simulink model "fullSystemModel"  (R2018a)
settings: Solver=ode3  StartTime=0.0  StopTime=1000  FixedStep=1  MinStep=1e-8  RelTol=1e-8
undefined symbols (not defined in the file or in its folder): DiscIntNeverNeededParam
libraries: BupSimulinkLibraries x32, simulink_extras x22, simulink x2, SignalEditorBlockLib x2
(part 2 of 3)

== system fullSystemModel/Easy_reg1/DataAnalyzer/InternalTrackingCourse ==
  Position : Inport  OutDataTypeStr=double  PortDimensions=3
  Azimuth : BupSimulinkLibraries/Azimuth
  Bearing : BupSimulinkLibraries/Bearing
  Display : Display
  Display1 : Display
  LastPos : Delay  DelayLength=1
  Manual Switch2 : ManualSwitch
  Radians to Degrees1 : simulink_extras/Transformations/Radians to Degrees
  Radians to Degrees2 : simulink_extras/Transformations/Radians to Degrees
  Scope1 : Scope  NumInputPorts=2
  Scope8 : Scope
  Scope9 : Scope
  Course : Outport  OutDataTypeStr=double  PortDimensions=1
  wires:
  Bearing/1 -> Manual Switch2/1, Display/1, Radians to Degrees1/1, Scope8/1
  Azimuth/1 -> Manual Switch2/2, Scope9/1, Radians to Degrees2/1, Display1/1
  Manual Switch2/1 -> Course/1
  LastPos/1 -> Azimuth/2, Bearing/2
  Position/1 -> LastPos/1, Bearing/1, Azimuth/1
  Radians to Degrees1/1 -> Scope1/1
  Radians to Degrees2/1 -> Scope1/2

== system fullSystemModel/Easy_reg1/DataAnalyzer/InternalTrackingSpeed ==
  Position : Inport
  Constant : Constant
  GPSVelocity : BupSimulinkLibraries/GPSVelocity
  LastPos1 : Delay  DelayLength=1
  ProjectionSpeed : BupSimulinkLibraries/ProjectionSpeed
  Hor_Velocity : Outport
  Ver_Velocity : Outport  Port=2
  wires:
  LastPos1/1 -> GPSVelocity/2
  ProjectionSpeed/2 -> Ver_Velocity/1
  Position/1 -> LastPos1/1, GPSVelocity/1
  ProjectionSpeed/1 -> Hor_Velocity/1
  GPSVelocity/1 -> ProjectionSpeed/1
  GPSVelocity/2 -> ProjectionSpeed/2
  GPSVelocity/3 -> ProjectionSpeed/3
  Constant/1 -> GPSVelocity/3

== system fullSystemModel/Easy_reg1/Targeting/Roughening ==
  Input : Inport
  DeadZone : BupSimulinkLibraries/DeadZone
  Gain : Gain  Gain=0.1
  Gain1 : Gain  Gain=10
  Manual Switch : ManualSwitch  CurrentSetting=0
  Rounding Function : Rounding
  Scope : Scope  NumInputPorts=3
  Output : Outport
  wires:
  Input/1 -> Scope/1, Gain/1
  Gain/1 -> Rounding Function/1
  Rounding Function/1 -> Gain1/1
  Gain1/1 -> Manual Switch/2, DeadZone/1, Scope/2
  DeadZone/1 -> Manual Switch/1, Scope/3
  Manual Switch/1 -> Output/1

== system fullSystemModel/Plant/GNSS/InternalTrackingCourse ==
  Position : Inport  OutDataTypeStr=double  PortDimensions=3
  Azimuth : BupSimulinkLibraries/Azimuth
  Bearing : BupSimulinkLibraries/Bearing
  Display : Display
  Display1 : Display
  LastPos : Memory  InheritSampleTime=on
  Manual Switch2 : ManualSwitch  CurrentSetting=0
  Scope1 : Scope  NumInputPorts=2
  Scope8 : Scope
  Scope9 : Scope
  Course : Outport  OutDataTypeStr=double  PortDimensions=1
  wires:
  Bearing/1 -> Scope1/1, Display/1, Manual Switch2/1, Scope8/1
  Azimuth/1 -> Display1/1, Scope1/2, Manual Switch2/2, Scope9/1
  Manual Switch2/1 -> Course/1
  LastPos/1 -> Azimuth/2, Bearing/2
  Position/1 -> LastPos/1, Bearing/1, Azimuth/1

== system fullSystemModel/Plant/GNSS/InternalTrackingCourse1 ==
  Position : Inport  OutDataTypeStr=double  PortDimensions=3
  Azimuth : BupSimulinkLibraries/Azimuth
  Bearing : BupSimulinkLibraries/Bearing
  Display : Display
  Display1 : Display
  LastPos : Memory  InheritSampleTime=on
  Manual Switch2 : ManualSwitch  CurrentSetting=0
  Scope1 : Scope  NumInputPorts=2
  Scope8 : Scope
  Scope9 : Scope
  Course : Outport  OutDataTypeStr=double  PortDimensions=1
  wires:
  Bearing/1 -> Scope1/1, Display/1, Manual Switch2/1, Scope8/1
  Azimuth/1 -> Display1/1, Scope1/2, Manual Switch2/2, Scope9/1
  Manual Switch2/1 -> Course/1
  LastPos/1 -> Azimuth/2, Bearing/2
  Position/1 -> LastPos/1, Bearing/1, Azimuth/1

== system fullSystemModel/Plant/GNSS/TrackingSpeed ==
  Position : Inport
  Constant : Constant
  GPSVelocity : BupSimulinkLibraries/GPSVelocity
  LastPos : Memory  InheritSampleTime=on  LinearizeAsDelay=on
  Vel_Latitude : Outport
  Vel_Longitude : Outport  Port=2
  Vel_Altitude : Outport  Port=3
  wires:
  LastPos/1 -> GPSVelocity/2
  Position/1 -> GPSVelocity/1, LastPos/1
  Constant/1 -> GPSVelocity/3
  GPSVelocity/3 -> Vel_Altitude/1
  GPSVelocity/2 -> Vel_Longitude/1
  GPSVelocity/1 -> Vel_Latitude/1

== system fullSystemModel/Plant/GNSS/Transformation ==
  InitialPos : Inport
  x : Inport  Port=2
  y : Inport  Port=3
  Bus Selector : BusSelector  OutputSignals=Initial_lat,Initial_lon
  Degrees to Radians : simulink_extras/Transformations/Degrees to Radians
  Divide : Product  Inputs=*/
  Gain : Gain  Gain=1/1000
  Gain1 : Gain  Gain=1/1000
  Gain5 : Gain  Gain=360/40000
  Gain6 : Gain  Gain=360/40000
  Sum : Sum  Inputs=++|
  Sum1 : Sum  Inputs=|++
  Trigonometric Function2 : Trigonometry  Operator=cos
  Latitude : Outport
  Longitude : Outport  Port=2
  wires:
  Divide/1 -> Sum1/1
  Gain5/1 -> Divide/1
  y/1 -> Gain1/1
  Gain6/1 -> Sum/1
  x/1 -> Gain/1
  Trigonometric Function2/1 -> Divide/2
  Degrees to Radians/1 -> Trigonometric Function2/1
  Gain/1 -> Gain5/1
  Gain1/1 -> Gain6/1
  InitialPos/1 -> Bus Selector/1
  Bus Selector/1 -> Sum/2  "<Initial_lat>"
  Bus Selector/2 -> Sum1/2  "<Initial_lon>"
  Sum/1 -> Degrees to Radians/1, Latitude/1
  Sum1/1 -> Longitude/1

== system fullSystemModel/Plant/GNSS/Transformation1 ==
  InitialPos : Inport
  x : Inport  Port=2
  y : Inport  Port=3
  Bus Selector : BusSelector  OutputSignals=Initial_lat,Initial_lon
  Degrees to Radians : simulink_extras/Transformations/Degrees to Radians
  Divide : Product  Inputs=*/
  Gain : Gain  Gain=1/1000
  Gain1 : Gain  Gain=1/1000
  Gain5 : Gain  Gain=360/40000
  Gain6 : Gain  Gain=360/40000
  Sum : Sum  Inputs=++|
  Sum1 : Sum  Inputs=|++
  Trigonometric Function2 : Trigonometry  Operator=cos
  Latitude : Outport
  Longitude : Outport  Port=2
  wires:
  Sum1/1 -> Longitude/1
  Sum/1 -> Latitude/1, Degrees to Radians/1
  Bus Selector/2 -> Sum1/2  "<Initial_lon>"
  Bus Selector/1 -> Sum/2  "<Initial_lat>"
  InitialPos/1 -> Bus Selector/1
  Gain1/1 -> Gain6/1
  Gain/1 -> Gain5/1
  Degrees to Radians/1 -> Trigonometric Function2/1
  Trigonometric Function2/1 -> Divide/2
  x/1 -> Gain/1
  Gain6/1 -> Sum/1
  y/1 -> Gain1/1
  Gain5/1 -> Divide/1
  Divide/1 -> Sum1/1

== system fullSystemModel/Plant/WindCreator/RotateOnNorth ==
  AbsoluteAngle : Inport
  Constant : Constant  Value=90
  Gain : Gain  Gain=-1
  Sum3 : Sum  Inputs=|+-
  OrientedOnNorth : Outport
  wires:
  AbsoluteAngle/1 -> Sum3/1
  Constant/1 -> Sum3/2
  Sum3/1 -> Gain/1
  Gain/1 -> OrientedOnNorth/1

== system fullSystemModel/flightController/DataAnalyzer/InternalTrackingCourse ==
  Position : Inport  OutDataTypeStr=double  PortDimensions=3
  Azimuth : BupSimulinkLibraries/Azimuth
  Bearing : BupSimulinkLibraries/Bearing
  Display : Display
  Display1 : Display
  LastPos : Delay  DelayLength=1
  Manual Switch2 : ManualSwitch
  Radians to Degrees1 : simulink_extras/Transformations/Radians to Degrees
  Radians to Degrees2 : simulink_extras/Transformations/Radians to Degrees
  Scope1 : Scope  NumInputPorts=2
  Scope8 : Scope
  Scope9 : Scope
  Course : Outport  OutDataTypeStr=double  PortDimensions=1
  wires:
  Bearing/1 -> Manual Switch2/1, Display/1, Radians to Degrees1/1, Scope8/1
  Azimuth/1 -> Manual Switch2/2, Scope9/1, Radians to Degrees2/1, Display1/1
  Manual Switch2/1 -> Course/1
  LastPos/1 -> Azimuth/2, Bearing/2
  Position/1 -> LastPos/1, Bearing/1, Azimuth/1
  Radians to Degrees1/1 -> Scope1/1
  Radians to Degrees2/1 -> Scope1/2

== system fullSystemModel/flightController/DataAnalyzer/InternalTrackingSpeed ==
  Position : Inport
  ExternalVelocity : Inport  Port=2
  Bus Selector1 : BusSelector  OutputSignals=gpsVelocity:latitude,gpsVelocity:longitude,gpsVelocity:altitude
  Constant : Constant
  GPSVelocity : BupSimulinkLibraries/GPSVelocity
  LastPos1 : Delay  DelayLength=1
  ProjectionSpeed : BupSimulinkLibraries/ProjectionSpeed
  Terminator : Terminator
  Terminator1 : Terminator
  Terminator2 : Terminator
  Hor_Velocity : Outport
  Ver_Velocity : Outport  Port=2
  wires:
  LastPos1/1 -> GPSVelocity/2
  ProjectionSpeed/2 -> Ver_Velocity/1
  Position/1 -> LastPos1/1, GPSVelocity/1
  ProjectionSpeed/1 -> Hor_Velocity/1
  Constant/1 -> GPSVelocity/3
  ExternalVelocity/1 -> Bus Selector1/1
  Bus Selector1/1 -> ProjectionSpeed/1  "<gpsVelocity:latitude>"
  Bus Selector1/2 -> ProjectionSpeed/2  "<gpsVelocity:longitude>"
  Bus Selector1/3 -> ProjectionSpeed/3  "<gpsVelocity:altitude>"
  GPSVelocity/1 -> Terminator/1
  GPSVelocity/2 -> Terminator1/1
  GPSVelocity/3 -> Terminator2/1

== system fullSystemModel/flightController/Targeting/Roughening ==
  Input : Inport
  DeadZone : BupSimulinkLibraries/DeadZone
  Gain : Gain  Gain=0.1
  Gain1 : Gain  Gain=10
  Manual Switch : ManualSwitch
  Rounding Function : Rounding
  Scope : Scope  NumInputPorts=3
  Output : Outport
  wires:
  Gain/1 -> Rounding Function/1
  Rounding Function/1 -> Gain1/1
  Gain1/1 -> Manual Switch/2, DeadZone/1, Scope/2
  DeadZone/1 -> Manual Switch/1, Scope/3
  Manual Switch/1 -> Output/1
  Input/1 -> Scope/1, Gain/1

== stateflow chart fullSystemModel/flightController/LogicController ==
  state Timer [parallel]
    entry:
    time = 0;
    BimSupply.timeout = 0;
    Control.Flight.StepAngle.timeout = 0;
    during:
    time = time + 1;
    BimSupply.timeout = TimeoutDecrement(BimSupply.timeout);
    Control.Flight.StepAngle.timeout = TimeoutDecrement(Control.Flight.StepAngle.timeout);
    settings: executionOrder=1
  state Control [parallel]
    % Основной цикл задач
    settings: executionOrder=2
    state Init % Производим планирование путевых точек для сброса высоты
      entry:
      targetPoint = touchdownPoint;
      %[Flight.Angle.Point1, Flight.Angle.Point2] = AngleManCreator(currentPoint, touchdownPoint, AngleManevr);
      %[Flight.Box.LUPoint, Flight.Box.LDPoint, Flight.Box.RUPoint, Flight.Box.RDPoint] = BOXCreator(touchdownPoint, BoxSize);
      Control.Flight.StepAngle.justReturnedHere = false;
      Control.Flight.StepAngle.waiting = true;
      initialPoint = currentPoint;
      touchdownPoint_Offset = [0;0;0];
    state TDP_Only % Режим прицеливания на TDP
      targetPoint = touchdownPoint;
      courseToTargetPoint = Azimut(targetPoint, currentPoint);
      %courseToTargetPoint = Heading(targetPoint, currentPoint, 0);
      desiredCourse = courseToTargetPoint;
    state Flight % Режим полета по точкам
      courseToTargetPoint = Azimut(targetPoint + touchdownPoint_Offset, currentPoint);
      %courseToTargetPoint = Heading(targetPoint + touchdownPoint_Offset, currentPoint, 0);
      desiredCourse = courseToTargetPoint;
      (history)
      state StepAngle
        coeff = nonlinearCoefficientFunction;
        timeDifference = timeVertical - timeHorizontal;
        state Right
          entry:
          timeout = uint32((timeDifference)*coeff)
          waiting = false;
          justReturnedHere = false;
          BimSupply.wantEnable;
          during:
          desiredCourse = Angle2Course(desiredCourse+AngleManevr);
          exit:
          if wherePoint(initialPoint, touchdownPoint, currentPoint) == -1
          side = false;
          else
          side = true;
          end
        state Wait
          entry:
          BimSupply.wantEnable
          waiting = true;
          justReturnedHere = true;
          exit:
          centralCourse = course;
        state Left
          entry:
          timeout = uint32((timeDifference)*coeff)
          waiting = false;
          justReturnedHere = false;
          BimSupply.wantEnable;
          during:
          desiredCourse = Angle2Course(desiredCourse-AngleManevr);
          exit:
          side = true;
          if wherePoint(initialPoint, touchdownPoint, currentPoint) == 1
          side = true;
          else
          side = false;
          end
        state Exit
        Right -> (junction 627) [order 2] : [errorCourseLimit]
            | {timeout = AngleTimeout/2;}
        Right -> (junction 627) [order 1] : [timeout == 0]
            | {timeout = AngleTimeout;}
        (default) -> Wait : {timeout = 15;}
        (junction 627) -> Wait
        Right -> (junction 627) [commented out] : Final
            | {timeout = AngleTimeout/2;}
        (junction 583) -> Right [order 1] : [side]
        Wait -> (junction 583) [order 1] : [(timeDifference) > 1  && timeout == 0]
        (junction 583) -> Left [order 2] : [~side]
        (default) -> Wait [commented out]
        Wait -> Exit [order 2] : [distanceToTarget < 500]
        Left -> (junction 624) [order 1] : [timeout == 0]
            | {timeout = AngleTimeout;}
        (junction 624) -> Wait
        Left -> (junction 624) [commented out] : Final
            | {timeout = AngleTimeout/2;}
        Left -> (junction 624) [order 2] : [errorCourseLimit]
            | {timeout = AngleTimeout/2;}
      state Angle % Режим углового манёвра [commented out]
        entry:
        targetPoint = EntryAngleMan (Point1, Point2, currentPoint, course);
      state Box [commented out]
        % LU - Нацеливание на верхний левый угол "коробки"
        % LD - Нацеливание на нижний левый угол "коробки"
        % RD - Нацеливание на нижний правый угол "коробки"
        % RU - Нацеливание на верхний правый угол "коробки"
        (history)
        state Init [commented out]
          BoxEntry = VerticeSelect(currentPoint, LUPoint, LDPoint, RUPoint, RDPoint);
        state RU [commented out]
          entry:
          targetPoint = RUPoint;
        state LU [commented out]
          entry:
          targetPoint = LUPoint;
        state LD [commented out]
          entry:
          targetPoint = LDPoint;
        state RD [commented out]
          entry:
          targetPoint = RDPoint;
        (default) -> Control.Flight.Box.Init [commented out]
        Control.Flight.Box.Init -> (junction 247) [commented out]
        (junction 247) -> RU [commented out] : [BoxEntry == 3]
        RU -> LU [commented out] : NextStage
        (junction 247) -> LU [commented out] : [BoxEntry == 1]
        LU -> LD [commented out] : NextStage
        RD -> RU [commented out] : NextStage
        (junction 247) -> RD [commented out] : [BoxEntry == 4]
        (junction 247) -> LD [commented out] : [BoxEntry == 2]
        LD -> RD [commented out] : NextStage
      state Final [commented out]
        % Состояние последнего манёвра
        % Цель которого выйти на заданную
        % точку приземления
        BimSupply.wantEnable;
        targetPoint = touchdownPoint
      note: Разрешаем обратные переходы,
          | но с таймаутом, чтобы избежать
          | лишних  переключений
      (default) -> (junction 265)
      (junction 265) -> StepAngle : [Mode == 2]
      (junction 265) -> Angle % Режим углового манёвра [commented out] : [Mode == 2]
      (junction 265) -> Box [commented out] : [Mode == 1]
      StepAngle -> Final [commented out] : final
      Angle % Режим углового манёвра -> Final [commented out] : final
      Angle % Режим углового манёвра -> Box [commented out] : nextStage
      Final -> Box [commented out] : cancelFinal
      Box -> Final [commented out] : final
    (default) -> Init % Производим планирование путевых точек для сброса высоты
    Init % Производим планирование путевых точек для сброса высоты -> (junction 168)
    (junction 168) -> TDP_Only % Режим прицеливания на TDP [order 1] : [Mode == 0]
    (junction 168) -> Flight % Режим полета по точкам [order 2] : [(Mode == 1 || Mode == 2) ]
  state Touchdown [parallel]
    %Здесь мы отдельно будем контролировать высоту,
    % для своевременного открытия посадотчных парашютов
    settings: executionOrder=3
    state On
      touchdownEnable = 1;
    state Off
      touchdownEnable = 0;
    (default) -> Off
    (junction 124) -> On : [(currentPoint(altitude)-reliefc) <= touchdownPoint(altitude)]
    (junction 122) -> On : [currentPoint(altitude) <= touchdownPoint(altitude)]
    Off -> (junction 118)
    (junction 118) -> (junction 122) [order 1] : [reliefAvailable == 0]
    (junction 118) -> (junction 124) [order 2] : [reliefAvailable ==1]
  state Timeoutput = TimeoutDecrement (TimeoutTag) [function]
    (default) -> (junction 574)
    (junction 574) -> (junction 575) [order 1] : [TimeoutTag > 0]
        | {Timeoutput = TimeoutTag - 1;}
    (junction 574) -> (junction 575) [order 2] : {Timeoutput = uint32(0);}
  state EventGenerator [parallel]
    entry:
    timeVertical = 0;
    timeHorizontal = 0;
    during:
    % Контроль выхода на точку
    if checkFinalMane  == 1;
    Control.final;
    else
    Control.cancelFinal;
    end
    % Контроль попадания в зону текущей цели
    if CheckArrival(currentPoint, targetPoint, ArrivalRadius) == 1;
    Control.nextStage;
    end
    % Контроль попадания в зону точки приземления
    % где на работу БИМов нет ограничений
    if CheckArrival(currentPoint, touchdownPoint, 2000) == 1;
    BimSupply.nonBlockingMode;
    BimTimeout = 10;
    end
    % Контроль попадания в зону точки приземления
    % Где управление уже запрещено
    if CheckArrival(currentPoint, touchdownPoint, 300) == 1;
    BimSupply.parking;
    end
    if fallingBim  == 1
    if Control.Flight.StepAngle.justReturnedHere
    Control.Flight.StepAngle.justReturnedHere = false;
    else
    BimSupply.wantDisable
    end
    end
    settings: executionOrder=4
  note: Final - Необходимость
      | перенацелиться
      | на точку приземления
      |
      | NextStage - Изменение
      | целевой точки на следу-
      | ющую, согласно алгоритму
      |
      | CancelFinal - На точку
      | приземления выходить
      | рано, высота избыточна
      |
      | if EndOfCorrection --->>>
      | Это условие даёт таймаут бимам с удержанием в нуле по падающему фронту команды. Но далее возникла необходимость, отличать такие фронты:
      | Фронт окончания настройки на TDP;
      | Фронт завершения манёвра понижения;
      | чтобы после манёвра понижения гарантированно сразу же разворачиваться на точку, а после уже можно дать таймаут.
      | justReturnedHere - Флаг, сообщающий о том, что алгоритм понижения только вернулся в состояние Wait;
  note: Входы:
      | touchdownPoint - Координаты точки приземления;
      | currentPoint - Текущие координаты;
      | reliefAvailable - Доступность карты рельефа местности (0 -недоступна, 1 - доступна);
      | reliefOnTDP - Высота рельефа над точкой приземления;
      | relief - Высота рельефа в текущем местоположении;
      | course - Путевой курс;
      | velocityHorizontal - Горизонтальная скорость полета по спутнику;
      | velocityVertical - Вертикальня скорость (снижения) по спутнику;
      | risingBim - Триггер по переднему фронту команды БИМам;
      | fallingBim - Триггер по падающему фронту команды БИМам;
      | touchdownPointOffset - Поправка к координатам точки приземления с учетом ветра;
  note: Выходы:
      | distanceToTarget - Горизонтальное расстояние до точки приземления, м;
      | timeHorizontal - Время горизонтального полета до точки приземления, сек;
      | timeVertical - Время вертикального полета до точки приземления, сек;
      | touchdownEnable - Команда на посадку;
      | enableTargetting - Разрешение/запрет работы БИМ;
      | desiredCourse - Желаемый курс полета;
      | skipOfSetSolution - Пропуск решения подсистемы определения ветра;
  note: Локальные:
      | targetPoint - Координаты пункта назначения;
      | touchdownPoint_Offset - Поправка на координаты пункта назначения с учетом влияния ветра;
      | initialPoint - Первая полученная координата, начало вектора ЛЗП;
      | centralCourse - Курс от которого откладывается угловой маневр потери высоты;
      | courseToTargetPoint - Курс до пункта назначения;
      | timeDifference - Разность времени горизонтального и вертикального полета
      |
      | Timer.time - Системное время;
      |
      | BimSupply.timeout - Таймаут на управление БИМами;
      | BimSupply.wantEnable - Входящее событие на включение БИМ;
      | BimSupply.wantDisable - Входящее событие на блокировку работы БИМ;
      | BimSupply.parking - Входящее событие на окончательное отключение БИМ;
      | BimSupply.nonBlockingMode - Входящее событие на переход в режим неблокируемого таймаутами режима работы БИМ;
      |
      | Control.final - Входящее событие завершения полета;
      | Control.cancelFinal - Входящее событие возврат из состояния завершения полета;
      | Control.nextStage - Прибытие в точку targetPoint;
      |
      | Control.Flight.StepAngle.justReturnedHere - Флаг-триггер подсистема переходит в состояние Wait;
      | Control.Flight.StepAngle.waiting - Флаг состояния подсистемы потери высоты (true - простаивает, false - в процессе манёвра);
      | Control.Flight.StepAngle.side - Флаг выбора стороны углового манёвра;
      | Control.Flight.StepAngle.coeff - Коэффициент эффективности уголового манёвра;
      | Control.Flight.StepAngle.timeout - Таймаут на угловые манёвры;
  state BimSupply [parallel]
    settings: executionOrder=5
    state Init
      entry:
      enableTargetting = 0;
    state Disable
      entry:
      enableTargetting = 0;
      timeout = BimTimeout;
    state Enable
      entry:
      timeout = 0;
      enableTargetting = 1;
    state NonBlockingControl [commented out]
      enableTargetting = 1;
    state Shutdown
      enableTargetting = 0;
    (default) -> BimSupply.Init
    Enable -> Disable [order 1] : wantDisable
    BimSupply.Init -> Enable
    Disable -> (junction 620) [order 2] : wantEnable
    Disable -> (junction 620) [order 3] : [timeout == 0]
    Disable -> NonBlockingControl [commented out] : nonBlockingMode
    Disable -> Shutdown [order 1] : parking
    Enable -> Shutdown [order 2] : parking
    Enable -> NonBlockingControl [commented out] : nonBlockingMode
    (junction 620) -> Enable
    NonBlockingControl -> Shutdown [commented out] : parking
  state OfsetTDP [parallel] [commented out]
    touchdownPoint_Offset = touchdownPointOffset;
    state Skip [commented out]
      skipOfsetSolution = true;
    state Get [commented out]
      skipOfsetSolution = false;
    (default) -> Get [commented out]
    Skip -> Get [commented out] : [Control.Flight.StepAngle.waiting]
    Get -> Skip [commented out] : [~Control.Flight.StepAngle.waiting]
  data: time local uint32 size=1; timeout local uint32 size=1; side local boolean size=1 =false; waiting local boolean size=1; coeff local double size=1; justReturnedHere local boolean size=1; Point1 local double size=3; Point2 local double size=3; LUPoint local double size=3; LDPoint local double size=3; RUPoint local double size=3; RDPoint local double size=3; BoxEntry local uint8 size=1; angle function_input; resultCourse function_output; TimeoutTag function_input uint32 size=1; Timeoutput function_output uint32 size=1; status function_output boolean size=1; coefficient function_output; status function_output; timeout local uint32 size=1; Mod local double size=3; skipNext local boolean size=1 =false; distanceToTarget output double size=1 =0; timeHorizontal output double size=1; timeVertical output double size=1; touchdownPoint input double size=4; currentPoint input double size=4; reliefAvailable input uint8 size=1; reliefc input int16 size=1; reliefOnTDP input int16 size=1; touchdownEnable output uint8 size=1; course input double size=1; BoxSize data_store_memory; ArrivalRadius data_store_memory; AngleManevr data_store_memory; Mode data_store_memory; velocityHorizontal input double size=1; velocityVertical input double size=1; TurnSpeed data_store_memory; fallingBim input boolean size=1; enableTargetting output uint8 size=1; desiredCourse output double size=1; targetPoint local double size=3; risingBim input boolean size=1; touchdownPointOffset input double size=3; BimTimeout data_store_memory; AngleTimeout data_store_memory; touchdownPoint_Offset local double size=3 =[0;0;0]; skipOfsetSolution output boolean size=1 =false; initialPoint local double size=3; centralCourse local double size=1; courseToTargetPoint local double size=1; timeDifference local double size=1; latitude constant uint8 =1; longitude constant uint8 =2; altitude constant uint8 =3; relief constant uint8 =4
  events: final local FUNCTION_CALL_EVENT; nextStage local FUNCTION_CALL_EVENT; cancelFinal local FUNCTION_CALL_EVENT; parking local FUNCTION_CALL_EVENT; nonBlockingMode local FUNCTION_CALL_EVENT; wantEnable local FUNCTION_CALL_EVENT; wantDisable local FUNCTION_CALL_EVENT
  function resultCourse = Angle2Course(angle):
    | %%%%%%%%%%%%%%%%%%%%%%%%%%%%%%%%%%%%%%%%%%%%%%%%%%%%%%%%%%%%%%%%%%%%%%%%%%%
    | % 
    | % Angle2Course - Преобразование курса к используемому в модели виду
    | %
    | %%%%%%%%%%%%%%%%%%%%%%%%%%%%%%%%%%%%%%%%%%%%%%%%%%%%%%%%%%%%%%%%%%%%%%%%%%%
    | function resultCourse = Angle2Course(angle)
    |     resultCourse = angle;
    |     if angle < 0
    |         resultCourse = resultCourse + 2*pi;
    |     end
    | end
  function status = checkFinalMane:
    | %%%%%%%%%%%%%%%%%%%%%%%%%%%%%%%%%%%%%%%%%%%%%%%%%%%%%%%%%%%%%%%%%%%%%%%%%%%
    | % CheckFinalMane - Проверка необходимости перехода к финальному манёвру
    | %%%%%%%%%%%%%%%%%%%%%%%%%%%%%%%%%%%%%%%%%%%%%%%%%%%%%%%%%%%%%%%%%%%%%%%%%%%
    | function status = checkFinalMane
    |     %% Вычислим расстояние с помощью функции DistanceCalculator()
    |     distanceToTarget = DistanceCalculator(currentPoint, touchdownPoint+touchdownPoint_Offset);
    |     %% Вычисляем время необходимое для преодоления расстояния до TDP и до посадки
    |     timeHorizontal = distanceToTarget/velocityHorizontal;
    |     timeVertical = (currentPoint(altitude) - (touchdownPoint(altitude) + double(reliefOnTDP)))/velocityVertical;
    |     %% Определяем поправку по времени необходимому на разворот
    |     % Угол разворота
    |     angle = ControlDemode(courseToTargetPoint - course);
    |     angle = abs(angle/pi*180);
    |     
    |     % Вычисляем поправку как линейную функцию: 
    |     %T_hor_popr = angle / TurnSpeed;
    | 
    |     % Вычисляем поправку по параболе
    |     timeHorizontalCorrection = 0.0005*angle^2 + 0.06*angle;
    |         
    |     % Нулевая поправка
    |     timeHorizontalCorrection = 0;
    |     
    |     timeHorizontal = timeHorizontal + timeHorizontalCorrection;
    |     %% Возвращаем сигнал о необходимости перейти на финальный маневр
    |     if timeHorizontal > timeVertical
    |         status = 1;
    |     else
    |         status = 0;
    |     end
    | end
  function coefficient = nonlinearCoefficientFunction:
    | %%%%%%%%%%%%%%%%%%%%%%%%%%%%%%%%%%%%%%%%%%%%%%%%%%%%%%%%%%%%%%%%%%%%%%%%%%%
    | %   nonlinearCoefficientFunction - Возвращает коэффициент эффективности
    | %   маневров потери высоты.
    | %%%%%%%%%%%%%%%%%%%%%%%%%%%%%%%%%%%%%%%%%%%%%%%%%%%%%%%%%%%%%%%%%%%%%%%%%%%
    | function coefficient = nonlinearCoefficientFunction()
    |     coefficient = 3*exp(-distanceToTarget/2.5e3);
    |     if coefficient > 1
    |         coefficient = 1;
    |     end
    | end
  function status = errorCourseLimit:
    | %%%%%%%%%%%%%%%%%%%%%%%%%%%%%%%%%%%%%%%%%%%%%%%%%%%%%%%%%%%%%%%%%%%%%%%%%%%
    | %   errorCourseLimit - Контролирует, чтобы при маневрах потери высоты,
    | %   разница курс до цели до начала маневра и после его завершения не были 
    | %   больше некоторого погового значения. Таким образом ограничиваем влияние
    | %   бокового ветра (не даём в боковом маневре уйти далеко от ЛЗП);
    | %%%%%%%%%%%%%%%%%%%%%%%%%%%%%%%%%%%%%%%%%%%%%%%%%%%%%%%%%%%%%%%%%%%%%%%%%%%
    | function status = errorCourseLimit()
    |     % centralCourse - курс до цели до начала манёвра
    |     result = abs(ControlDemode(courseToTargetPoint-centralCourse));
    |     if result > (25/180*pi)
    |         status = 1;
    |     else
    |         status = 0;
    |     end
    | end

== stateflow chart fullSystemModel/Easy_reg1/TaskController ==
  state Timer [parallel]
    entry:
    time = 0;
    during:
    time = time + 1;
    if BimSupply.timeout > 0
    BimSupply.timeout = BimSupply.timeout - 1;
    end
    settings: executionOrder=1
  state Control [parallel]
    % Основной цикл задач
    settings: executionOrder=2
    state Init % Производим планирование путевых точек для сброса высоты
      entry:
      TargetPoint = TDPoint;
      [Flight.Angle.Point1, Flight.Angle.Point2] = AngleManCreator(ActualPoint, TDPoint, AngleManevr);
      [Flight.Box.LUPoint, Flight.Box.LDPoint, Flight.Box.RUPoint, Flight.Box.RDPoint] = BOXCreator(TDPoint, BoxSize);
    state TDP_Only % Режим прицеливания на TDP
      %entry:
      TargetPoint = TDPoint;
    state Flight % Режим полета по точкам
      (history)
      state Angle % Режим углового манёвра
        entry:
        TargetPoint = EntryAngleMan (Point1, Point2, ActualPoint, Course);
      state Box
        % LU - Нацеливание на верхний левый угол "коробки"
        % LD - Нацеливание на нижний левый угол "коробки"
        % RD - Нацеливание на нижний правый угол "коробки"
        % RU - Нацеливание на верхний правый угол "коробки"
        (history)
        state Init
          BoxEntry = VerticeSelect(ActualPoint, LUPoint, LDPoint, RUPoint, RDPoint);
        state RU
          entry:
          TargetPoint = RUPoint;
        state LU
          entry:
          TargetPoint = LUPoint;
        state LD
          entry:
          TargetPoint = LDPoint;
        state RD
          entry:
          TargetPoint = RDPoint;
        (default) -> Init
        Init -> (junction 247)
        (junction 247) -> RU [order 4] : [BoxEntry == 3]
        (junction 247) -> LU [order 1] : [BoxEntry == 1]
        RU -> LU : NextStage
        (junction 247) -> LD [order 3] : [BoxEntry == 2]
        (junction 247) -> RD [order 2] : [BoxEntry == 4]
        LU -> LD : NextStage
        RD -> RU : NextStage
        LD -> RD : NextStage
      state Final
        % Состояние последнего манёвра
        % Цель которого выйти на заданную
        % точку приземления
        entry:
        TargetPoint = TDPoint;
      note: Разрешаем обратные переходы,
          | но с таймаутом, чтобы избежать
          | лишних  переключений
      (default) -> (junction 265)
      (junction 265) -> Box [order 1] : [Mode == 1]
      (junction 265) -> Angle % Режим углового манёвра [order 2] : [Mode == 2]
      Angle % Режим углового манёвра -> Final [order 2] : Final
      Angle % Режим углового манёвра -> Box [order 1] : NextStage
      Box -> Final : Final
      Final -> Box [commented out] : CancelFinal
          | [Timer.timeout == 0]
    (default) -> Init % Производим планирование путевых точек для сброса высоты
    Init % Производим планирование путевых точек для сброса высоты -> (junction 168)
    (junction 168) -> TDP_Only % Режим прицеливания на TDP [order 1] : [Mode == 0]
    (junction 168) -> Flight % Режим полета по точкам [order 2] : [(Mode == 1 || Mode == 2) ]
  note: Данный метод основан на предыдущем механизме прицеливания,
      | однако теперь с помощью Stateflow алгоритм управления будет
      | построен на полете по заданным точкам.
      | Таким образом необходимо организовать планирование полётных точек,
      | и способ их подстановки в мат.модель прицеливания.
  state TargetCourse [parallel]
    %Course2Target = Azimut(TargetPoint, ActualPoint);
    Course2Target = Heading(TargetPoint, ActualPoint, 0);
    settings: executionOrder=3
  state Simulink [group] [commented out]
    % Подсистемы из симулинк блоков
  state Touchdown [parallel]
    %Здесь мы отдельно будем контролировать высоту,
    % для своевременного открытия посадотчных парашютов
    settings: executionOrder=4
    state OFF
      TD_CMD = 0;
    state ON
      TD_CMD = 1;
    (default) -> OFF
    OFF -> (junction 118)
    (junction 124) -> ON : [(ActualPoint(3)-Relief) <= TDPoint(3)]
    (junction 122) -> ON : [ActualPoint(3) <= TDPoint(3)]
    (junction 118) -> (junction 122) [order 1] : [ReliefAvailable == 0]
    (junction 118) -> (junction 124) [order 2] : [ReliefAvailable ==1]
  state EventGenerator [parallel]
    during:
    % Контроль выхода на точку
    if func.CheckFinalMane  == 1;
    Control.Final;
    end
    % Контроль попадания в зону текущей цели
    if CheckArrival(ActualPoint, TargetPoint, ArrivalRadius) == 1;
    Control.NextStage;
    else
    Control.CancelFinal;
    end
    % Контроль попадания в зону точки приземления
    % где на работу БИМов нет ограничений
    if CheckArrival(ActualPoint, TDPoint, 1000) == 1;
    BimSupply.NonBlockingMode;
    end
    % Контроль попадания в зону точки приземления
    % Где управление уже запрещено
    if CheckArrival(ActualPoint, TDPoint, 300) == 1;
    BimSupply.Parking;
    end
    settings: executionOrder=5
  note: Final - Необходимость
      | перенацелиться
      | на точку приземления
      |
      | NextStage - Изменение
      | целевой точки на следу-
      | ющую, согласно алгоритму
      |
      | CancelFinal - На точку
      | приземления выходить
      | рано, высота избыточна
  state func [group]
    % Реализации всех m-функций
  state BimSupply [parallel]
    entry:
    timeout = 0;
    TargetEnable = 1;
    settings: executionOrder=6
    state Enable
      entry:
      TargetEnable = 1;
    state Disable
      entry:
      TargetEnable = 0;
      timeout = 30;
    state NonBlockingControl
      TargetEnable = 1;
    state Shutdown
      TargetEnable = 0;
    (default) -> Enable
    Enable -> Disable [order 2] : [EndOfCorrection  == 1]
    Enable -> NonBlockingControl [order 1] : NonBlockingMode
    Disable -> Enable [order 2] : [timeout == 0]
    Disable -> NonBlockingControl [order 1] : NonBlockingMode
    NonBlockingControl -> Shutdown : Parking
  data: time local uint32 size=1; Point1 local double size=3; Point2 local double size=3; LUPoint local double size=3; LDPoint local double size=3; RUPoint local double size=3; RDPoint local double size=3; BoxEntry local uint8 size=1; Initial_point function_input double size=3; TDP function_input double size=3; AMP1 function_output double size=3; AMP2 function_output double size=3; Angle function_input double size=3; TDP function_input size=3; BLU function_output size=3; BLD function_output size=3; BRU function_output size=3; BRD function_output size=3; BoxStep function_input size=1; InputPoint function_input size=3; OutputPoint function_output size=3; AMP function_input double size=3; BLU function_input double size=3; BLD function_input double size=3; BRU function_input double size=3; BRD function_input double size=3; Vertice function_output uint8 size=1; AM1 function_input double size=3; AM2 function_input double size=3; Position function_input double size=1; point function_output double size=1; TrackingCourse function_input double size=1; Position function_input size=3; Target function_input size=3; y function_output size=1; Now function_input double size=3; To function_input double size=3; status function_output boolean size=1; Radius function_input double size=1; status function_output boolean size=1; To function_input double size=3; From function_input double size=3; y function_output double size=1; timeout local uint32 size=1; Distance output double size=1; T_hor output double size=1; T_ver output double size=1; TDPoint input double size=3; ActualPoint input double size=3; ReliefAvailable input uint8 size=1; Relief input int16 size=1; ReliefOnTDP input int16 size=1; TD_CMD output uint8 size=1; Course input double size=1; BoxSize data_store_memory; ArrivalRadius data_store_memory; AngleManevr data_store_memory; Mode data_store_memory; V_hor input double size=1; V_ver input double size=1; TurnSpeed data_store_memory; Course2TDP input double size=1; EndOfCorrection input boolean size=1; TargetEnable output uint8 size=1; Course2Target output double size=1; TargetPoint local double size=3; StartOfCorrection input boolean size=1; TDPPopr input double size=3
  events: Final local FUNCTION_CALL_EVENT; NextStage local FUNCTION_CALL_EVENT; CancelFinal local FUNCTION_CALL_EVENT; Parking local FUNCTION_CALL_EVENT; NonBlockingMode local FUNCTION_CALL_EVENT
  function [AMP1, AMP2] = AngleManCreator(Initial_point, TDP, Angle):
    | %%%%%%%%%%%%%%%%%%%%%%%%%%%%%%%%%%%%%%%%%%%%%%%%%%%%%%%%%%%%%%%%%%%%%%%%%%%
    | % AngleManCreator - Создание точек углового манёвра по обе стороны от ЛЗП
    | %%%%%%%%%%%%%%%%%%%%%%%%%%%%%%%%%%%%%%%%%%%%%%%%%%%%%%%%%%%%%%%%%%%%%%%%%%%
    | function [AMP1, AMP2] = AngleManCreator(Initial_point, TDP, Angle)
    |     %% Расшифровка переменных
    |     % AMP - Координата углового манёвра
    |     %% Это точка углового манёвра расчитанная по равностороннему треугольнику
    |     x1 = Initial_point(2);
    |     y1 = Initial_point(1);
    |     x2 = TDP(2);
    |     y2 = TDP(1);
    |     % Возьмем половину расстояния до точки посадки и повернём этот вектор на
    |     dx = (x2-x1)/2;
    |     dy = (y2-y1)/2;
    |     % Определяем первую точку
    |     x3 = dx*cos(Angle*pi/180) - dy*sin(Angle*pi/180)+x1;
    |     y3 = dx*sin(Angle*pi/180) + dy*cos(Angle*pi/180)+y1;
    |     AMP1 = [y3;x3;0];
    |     % Определяем вторую точку
    |     x4 = dx*cos(-Angle*pi/180) - dy*sin(-Angle*pi/180)+x1;
    |     y4 = dx*sin(-Angle*pi/180) + dy*cos(-Angle*pi/180)+y1;
    |     AMP2 = [y4;x4;0];
    |     %% Проверим выход точек за пределы координат
    |     AMP1 = PositionRangeConverting(AMP1);
    |     AMP2 = PositionRangeConverting(AMP2);
    | end
  function [BLU, BLD, BRU, BRD] = BOXCreator(TDP, BoxStep):
    | %%%%%%%%%%%%%%%%%%%%%%%%%%%%%%%%%%%%%%%%%%%%%%%%%%%%%%%%%%%%%%%%%%%%%%%%%%%
    | % BOXCreator - Создание опорных точек аварийного манёвра "Коробка"
    | %%%%%%%%%%%%%%%%%%%%%%%%%%%%%%%%%%%%%%%%%%%%%%%%%%%%%%%%%%%%%%%%%%%%%%%%%%%
    | function [BLU, BLD, BRU, BRD] = BOXCreator(TDP, BoxStep)
    |     %% Расшифровка переменных
    |     % BLU - Координата верхней левой точки квадрата
    |     % BLD - Координата нижней левой точки квадрата
    |     % BRU - Координата верхней правой точки квадрата
    |     % BRD - Координата нижней правой точки квадрата
    |     %% Расчитываем точки квадрата
    |     BLU=[0; 0; 0]; BLD = [0; 0; 0]; BRU = [0; 0; 0]; BRD=[0; 0; 0];
    |     % Вычисляем шаг в градусах по Широте (однозначно сопоставляются)
    |     LatStep = BoxStep/1000*360/40000;
    |     % Координаты по Широте
    |     BLU(1) = TDP(1) + LatStep;
    |     BLD(1) = TDP(1) - LatStep; 
    |     BRU(1) = TDP(1) + LatStep;
    |     BRD(1) = TDP(1) - LatStep; 
    |     % Вычисляем шаг по Долготе без учета поправки на Широту (долгота зависит от
    |     % широты), а поправку на широту будем делать прямо в выражении
    |     LonStep = BoxStep/1000*360/40000;
    |     % Координаты по Долготе
    |     BLU(2) = TDP(2) - LonStep/cos(pi*BLU(1)/180);
    |     BLD(2) = TDP(2) - LonStep/cos(pi*BLD(1)/180);
    |     BRU(2) = TDP(2) + LonStep/cos(pi*BRU(1)/180);
    |     BRD(2) = TDP(2) + LonStep/cos(pi*BRD(1)/180);
    |     %% Проверим выход точек за пределы координат
    |     BLU = PositionRangeConverting(BLU);
    |     BLD = PositionRangeConverting(BLD);
    |     BRU = PositionRangeConverting(BRU);
    |     BRD = PositionRangeConverting(BRD);
    | end
  function OutputPoint = PositionRangeConverting(InputPoint):
    | %%%%%%%%%%%%%%%%%%%%%%%%%%%%%%%%%%%%%%%%%%%%%%%%%%%%%%%%%%%%%%%%%%%%%%%%%%%
    | % PositionRangeConverting - Проверка корректности сферических координат 
    | %%%%%%%%%%%%%%%%%%%%%%%%%%%%%%%%%%%%%%%%%%%%%%%%%%%%%%%%%%%%%%%%%%%%%%%%%%%
    | function OutputPoint = PositionRangeConverting(InputPoint)
    |     %% Контроль пределов Координат
    |     % InputPoint(1) - Широта
    |     % InputPoint(2) - Долгота
    |     % InputPoint(3) - Высота
    |     OutputPoint = InputPoint;
    |     %% Преобразование Долготы
    |     if OutputPoint(2) > 180
    |         OutputPoint(2) = OutputPoint(2) - 360;
    |     elseif OutputPoint(2) < (-180)
    |         OutputPoint(2) = OutputPoint(2) + 360;
    |     end
    | end
  function Vertice = VerticeSelect(AMP, BLU, BLD, BRU, BRD):
    | %%%%%%%%%%%%%%%%%%%%%%%%%%%%%%%%%%%%%%%%%%%%%%%%%%%%%%%%%%%%%%%%%%%%%%%%%%%
    | %  VerticeSelect - Выбор оптимального входа в манёвр "коробка"
    | %
    | %  AMP - Координаты точки, от которой расчитывается вход
    | %  BLU - Координаты точки левого верхнего угла коробки
    | %  BLD - Координаты точки левого нижнего угла коробки 
    | %  BRU - Координаты точки правого верхнего угла коробки 
    | %  BRD - Координаты точки нижнего верхнего угла коробки
    | %
    | %  Возвращает номер вершины оптимального входа
    | %      1 - BLU, 2 - BLD, 3 - BRU, 4 - BRD
    | %%%%%%%%%%%%%%%%%%%%%%%%%%%%%%%%%%%%%%%%%%%%%%%%%%%%%%%%%%%%%%%%%%%%%%%%%%%
    | function Vertice = VerticeSelect(AMP, BLU, BLD, BRU, BRD)
    |     %% Функция определения точки входа в "посадочной коробке"
    |     D_BLU = DistanceCalculator(AMP,BLU);
    |     D_BLD = DistanceCalculator(AMP,BLD);
    |     D_BRU = DistanceCalculator(AMP,BRU);
    |     D_BRD = DistanceCalculator(AMP,BRD);
    |     %% Соответсвие значения Vertice и вершин коробки
    |     % 1 - Левая верхняя
    |     % 2 - Левая нижняя
    |     % 3 - Правая верхняя
    |     % 4 - Правая нижняя
    |     x = [D_BLU, D_BLD, D_BRU, D_BRD]; 
    |     Vertice = 1;
    |     for i = 1:1:3
    |         if x(i+1) < x(Vertice)
    |             Vertice = i+1;
    |         end
    |     end
    |     Vertice = uint8(Vertice);
    | end
  function point = EntryAngleMan (AM1, AM2, Position, TrackingCourse):
    | %%%%%%%%%%%%%%%%%%%%%%%%%%%%%%%%%%%%%%%%%%%%%%%%%%%%%%%%%%%%%%%%%%%%%%%%%%%
    | % EntryAngleMan - Определение оптимальной точки входа в угловой манёвр
    | % AM1            - Точка углового манёвра 1
    | % AM2            - Точка углового манёвра 2
    | % Position       - Текущие координаты
    | % TrackingCourse - Текущий курс
    | %
    | % Возвращает одну из точек (AM1 или AM2) в зависимости от оптимальности
    | %%%%%%%%%%%%%%%%%%%%%%%%%%%%%%%%%%%%%%%%%%%%%%%%%%%%%%%%%%%%%%%%%%%%%%%%%%%
    | function point = EntryAngleMan (AM1, AM2, Position, TrackingCourse)
    |     %% Определим курс до точек манёвра
    |     Course1 = CourseCalculator(AM1, Position);
    |     Course2 = CourseCalculator(AM2, Position);
    |     %% Найдём разницу с путевым
    |     Course1 = Course1 - TrackingCourse;
    |     Course2 = Course2 - TrackingCourse;
    |     %% Проведем нормирование разницы
    |     if Course1 > pi
    |         Course1 = Course1 - 2*pi;
    |     end
    |     if Course1 < (-pi)
    |         Course1 = Course1 + 2*pi;
    |     end
    |     if Course2 > pi
    |         Course2 = Course2 - 2*pi;
    |     end
    |     if Course2 < (-pi)
    |         Course2 = Course2 + 2*pi;
    |     end
    |     %% Возьмём модуль для сравнения
    |     Course1 = abs(Course1);
    |     Course2 = abs(Course2);
    |     %% Будет выбрана точка до которой поворот меньше
    |     if Course1 < Course2
    |         point = AM1;
    |     else
    |         point = AM2;
    |     end
    | end
  function y = DistanceCalculator (Position, Target):
    | %%%%%%%%%%%%%%%%%%%%%%%%%%%%%%%%%%%%%%%%%%%%%%%%%%%%%%%%%%%%%%%%%%%%%%%%%%%
    | % DistanceCalculator - Вычисление расстрояния от Position до Target 
    | % в метрах по сферическим координатам
    | %%%%%%%%%%%%%%%%%%%%%%%%%%%%%%%%%%%%%%%%%%%%%%%%%%%%%%%%%%%%%%%%%%%%%%%%%%%
    | function y = DistanceCalculator (Position, Target)
    |     %% Вычитаем расстояние (через вектора)
    |     % dif = (TDP - ActualPoint);
    |     % % Вычисляем проекции на оси с переводом в Км.
    |     % distance_lon2x = dif(1)*40000/360*cos(dif(2)*pi/180);
    |     % distance_lat2y = dif(2)*40000/360;
    |     % distance = sqrt(distance_lon2x^2 + distance_lat2y^2);
    |     %% Вычитаем расстояние (через тригонометрию)
    |     la1 = Position(2)*pi/180;
    |     fi1 = Position(1)*pi/180;
    |     la2 = Target(2)*pi/180;
    |     fi2 = Target(1)*pi/180;
    |     d = sin(fi1)*sin(fi2) + cos(fi1)*cos(-fi2)*cos(la2-la1);
    |     % 6371 км средний радиус земли
    |     y = acos(d)*6371e3;
    | end
  function status = CheckArrival (Now, To, Radius):
    | %%%%%%%%%%%%%%%%%%%%%%%%%%%%%%%%%%%%%%%%%%%%%%%%%%%%%%%%%%%%%%%%%%%%%%%%%%%
    | % CheckArrival - Проверка прибытия в точку с координатами "To"
    | % Now    - Текущие координаты
    | % To     - Координаты точки приземления
    | % Radius - Радиус зоны попадания, м
    | %%%%%%%%%%%%%%%%%%%%%%%%%%%%%%%%%%%%%%%%%%%%%%%%%%%%%%%%%%%%%%%%%%%%%%%%%%%
    | function status = CheckArrival (Now, To, Radius)
    |     %% Вычитаем коррдинаты и берем модуль
    |     %dif = (To - Now);
    |     %distance = sqrt(dif(1)^2 + dif(2)^2);
    |     %% Вычисляем расстояние с помощью DistanceCalculator
    |     distance = DistanceCalculator (Now, To);
    |     %% Попаданием будем считать радиус 
    |     if distance < Radius
    |         status = 1;
    |     else
    |         status = 0;
    |     end
    | end
  function status = CheckFinalMane:
    | %%%%%%%%%%%%%%%%%%%%%%%%%%%%%%%%%%%%%%%%%%%%%%%%%%%%%%%%%%%%%%%%%%%%%%%%%%%
    | % CheckFinalMane - Проверка необходимости перехода к финальному манёвру
    | %
    | % Использует глобальные переменные:
    | %    ActualPoint - Текущие координаты
    | %    TDPoint     - Координаты точки приземления
    | %    V_hor       - Горизонтальная скорость полета (м/с)
    | %    V_ver       - Скорость снижения (м/c)
    | %    Course      - Путевой курс
    | %    Course2TDP  - Курс (азимут) до точки приземления
    | %    ReliefOnTDP - Высота рельефа над точкой приземления
    | %
    | %%%%%%%%%%%%%%%%%%%%%%%%%%%%%%%%%%%%%%%%%%%%%%%%%%%%%%%%%%%%%%%%%%%%%%%%%%%
    | function status = CheckFinalMane ()
    |     %% Вычислим расстояние с помощью функции DistanceCalculator()
    |     Distance = DistanceCalculator(ActualPoint, TDPoint);
    |     %% Вычисляем время необходимое для преодоления расстояния до TDP и до посадки
    |     T_hor = Distance/V_hor;
    |     T_ver = (ActualPoint(3) - (TDPoint(3) + double(ReliefOnTDP)))/V_ver;
    |     %% Определяем поправку по времени необходимому на разворот
    |     % Угол разворота
    |     angle = abs(Course2TDP-Course) * 180 / pi;
    |     if angle > 180
    |         angle = angle - 180;
    |     end
    | 
    |     % Вычисляем поправку как линейную функцию: 
    |     T_hor_popr = angle / TurnSpeed;
    | 
    |     % Вычисляем поправку по параболе
    |     %T_hor_popr = 0.003*angle^2 + 0.008*angle;
    | 
    |     T_hor = T_hor + T_hor_popr;
    |     %% Возвращаем сигнал о необходимости перейти на финальный маневр
    |     if T_hor > T_ver
    |         status = 1;
    |     else
    |         status = 0;
    |     end
    | end
  function y = CourseCalculator(To, From):
    | %%%%%%%%%%%%%%%%%%%%%%%%%%%%%%%%%%%%%%%%%%%%%%%%%%%%%%%%%%%%%%%%%%%%%%%%%%%
    | % CourseCalculator - Вычисление азимута от точки FROM до точки TO
    | %%%%%%%%%%%%%%%%%%%%%%%%%%%%%%%%%%%%%%%%%%%%%%%%%%%%%%%%%%%%%%%%%%%%%%%%%%%
    | function y = CourseCalculator(To, From)
    | %% Высчитаем, как изменились координаты
    | un = To - From;
    | d_lat = un(1);
    | d_lon = un(2);
    | %% Условие для определения кратчайшего пути с учетом переходов между
    | % меридианами 0 и 180 по долготе
    | if d_lon > 180
    |     d_lon = d_lon - 360;
    | elseif d_lon < (-180)
    |         d_lon = d_lon +360;
    | end
    | %% Расчет курса
    | un_pow1 = d_lat*d_lat;
    | un_pow2 = d_lon*d_lon;
    | if (un_pow1 < 1e-16) && (un_pow2 < 1e-16)
    |     y = 0;
    | else
    |     x = acos( d_lon / (sqrt(un_pow2 + un_pow1)));
    |     y = acos( d_lat / (sqrt(un_pow2 + un_pow1)));
    |     if x > 1.5708
    |         y = 6.28319 - y;
    |     end
    | end

== matlab function fullSystemModel/flightController/Targeting/MATLAB Function ==
  data: u input; y output
function y = fcn(u)
s = 5;
y = u;
if u < - s
    y = -50;
elseif u > s
    y = 50;
end
end

== stateflow chart fullSystemModel/flightController/Targeting/TimeNAngleTurning ==
  state Prepare
    entry:
    StrapSecond = 0;
    Error = 0;
    FixedStrapPosition = 0;
    StrapPosition = 0;
    during:
    Error = abs(AngleError);
    if Enable == 1
    if Error > 5
    StrapSecond = uint16(Error/(abs(StrapLimit)*TurnSpeed));
    FixedStrapPosition = StrapLimit;
    Action;
    end
    end
  state StrapAction
    entry:
    StrapPosition = FixedStrapPosition;
    during:
    if StrapSecond > 0
    StrapSecond = StrapSecond - 1;
    end
  (default) -> Prepare
  StrapAction -> Prepare [order 2] : [Enable == 0]
  StrapAction -> Prepare [order 1] : [StrapSecond == 0]
      | {StrapPosition = 0;}
  Prepare -> StrapAction : Action
  data: Enable input uint8 size=1; AngleError input double size=1; TurnSpeed input double size=1; StrapPosition output double size=1; FixedStrapPosition local double size=1; StrapSecond local uint16 size=1; StrapLimit input double size=1; Error local double size=1
  events: Action local FUNCTION_CALL_EVENT

== stateflow chart fullSystemModel/flightController/feedback/Chart ==
  state Initialization
    initialGroundSpeed = 0;
    initialCourse = 0;
    currentGroundSpeed = 0;
    currentCourse = 0;
    windForce = 0;
    windCourse = 0;
  state FixInitialVector
    entry:
    initialGroundSpeed = groundSpeed;
    initialCourse = course;
  state GetResult
    entry:
    [windForce, windCourse] = WindEstimator(initialGroundSpeed, initialCourse, currentGroundSpeed, currentCourse, 20)
    initialGroundSpeed = currentGroundSpeed;
    initialCourse = currentCourse;
  state Pause
  state FixCurrentVector
    entry:
    currentGroundSpeed = groundSpeed;
    currentCourse = course;
  (default) -> Initialization
  Initialization -> FixInitialVector : [bimWasEnabled == 1]
  FixInitialVector -> (junction 37)
  GetResult -> (junction 37)
  (junction 37) -> Pause : [bimWasDisabled == 1]
  Pause -> FixCurrentVector : [bimWasEnabled == 1]
  FixCurrentVector -> GetResult
  data: bimWasEnabled input boolean size=1; bimWasDisabled input boolean size=1; initialGroundSpeed local double size=1; currentGroundSpeed local double size=1; initialCourse local double size=1; currentCourse local double size=1; groundSpeed input double size=1; course input double size=1; windForce output double size=1; windCourse output double size=1; airSpeed input double size=1; timeHasPassed local uint32 size=1
